simulink model "Res_Angle_Const"  (Simulink 7.6)
settings: Solver=ode45  StartTime=0.0  StopTime=0.02  RelTol=1e-3
settings Model: Creator=Vano  LastModifiedBy=Vano

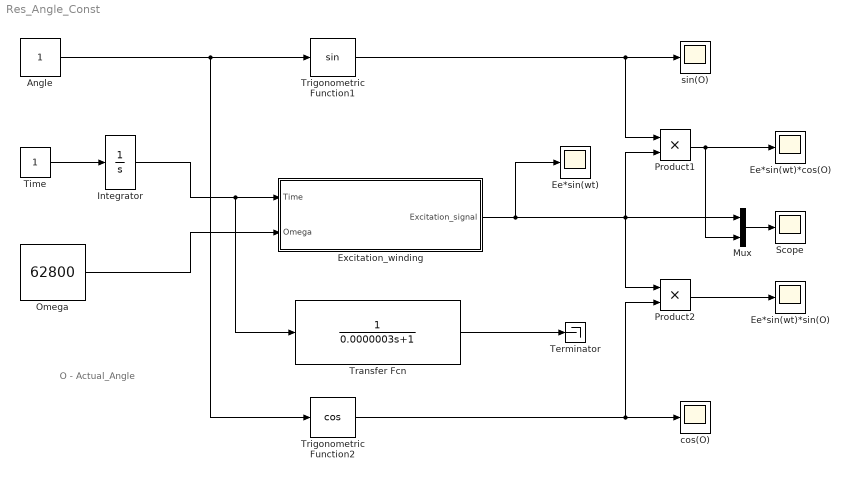
== system Res_Angle_Const ==
  note: O - Actual_Angle
  Angle : Constant
  Ee*sin(wt) : Scope
      settings: SaveName=ScopeData2
  Ee*sin(wt)*cos(O) : Scope
  Ee*sin(wt)*sin(O) : Scope
      settings: SaveName=ScopeData3
  Excitation_winding : Subsystem
  Integrator : Integrator
  Mux : Mux  Inputs=2
  Omega : Constant  Value=62800
  Product1 : Product  RndMeth=Zero
  Product2 : Product  RndMeth=Zero
  Scope : Scope
      settings: SaveName=ScopeData5
  Terminator : Terminator
  Time : Constant
  Transfer Fcn : TransferFcn  Denominator=[0.0000003 1]
  Trigonometric Function1 : Trigonometry
  Trigonometric Function2 : Trigonometry  Operator=cos
  cos(O) : Scope
      settings: SaveName=ScopeData4
  sin(O) : Scope
  wires:
  Time/1 -> Integrator/1
  Omega/1 -> Excitation_winding/2(Omega)
  Integrator/1 -> Transfer Fcn/1, Excitation_winding/1(Time)
  Trigonometric Function1/1 -> sin(O)/1, Product1/1
  Excitation_winding/1(Excitation_signal) -> Product2/1, Product1/2, Mux/1, Ee*sin(wt)/1
  Trigonometric Function2/1 -> Product2/2, cos(O)/1
  Product1/1 -> Ee*sin(wt)*cos(O)/1, Mux/2
  Product2/1 -> Ee*sin(wt)*sin(O)/1
  Transfer Fcn/1 -> Terminator/1
  Mux/1 -> Scope/1
  Angle/1 -> Trigonometric Function1/1, Trigonometric Function2/1

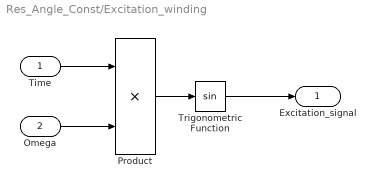
== system Res_Angle_Const/Excitation_winding ==
  Time : Inport
  Omega : Inport  Port=2
  Product : Product  RndMeth=Zero
  Trigonometric Function : Trigonometry
  Excitation_signal : Outport
  wires:
  Product/1 -> Trigonometric Function/1
  Time/1 -> Product/1
  Trigonometric Function/1 -> Excitation_signal/1
  Omega/1 -> Product/2
